simulink model "TP03"  (R2023a)
settings: Solver=ode45  StartTime=0.0  StopTime=2  FixedStep=5  RelTol=1e-3
undefined symbols (not defined in the file): DiscIntNeverNeededParam, K, ue, x0, xe
libraries: simulink x1
settings Model: Creator=pmt1554  LastModifiedBy=pmt1554

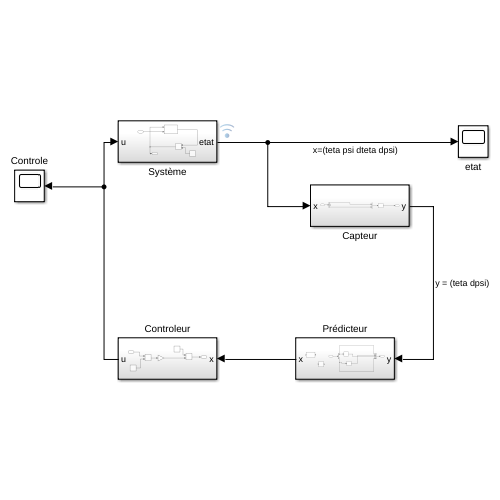
[thumbnail: Simulink's stored preview of the top-level diagram]
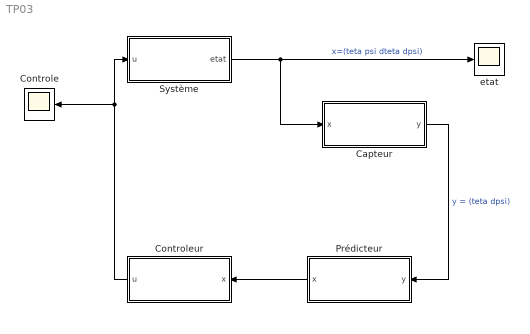
== system TP03 ==
  Capteur : Subsystem
  Controle : Scope
  Controleur : Subsystem
  Prédicteur : Subsystem
  Système : Subsystem
  etat : Scope
  wires:
  Système/1(etat) -> Capteur/1(x), etat/1  "x=(teta psi dteta dpsi)"
  Controleur/1(u) -> Système/1(u), Controle/1
  Capteur/1(y) -> Prédicteur/1(y)  "y = (teta dpsi)"
  Prédicteur/1(x) -> Controleur/1(x)

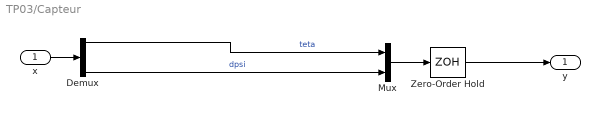
== system TP03/Capteur ==
  x : Inport
  Demux : Demux
  Mux : Mux  Inputs=2
  Zero-Order Hold : ZeroOrderHold  SampleTime=0.001
  y : Outport
  wires:
  x/1 -> Demux/1
  Mux/1 -> Zero-Order Hold/1
  Demux/1 -> Mux/1  "teta"
  Demux/4 -> Mux/2  "dpsi"
  Zero-Order Hold/1 -> y/1

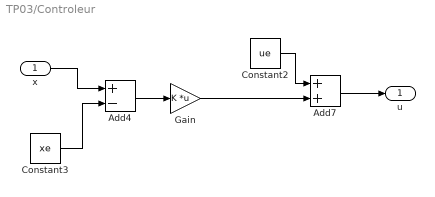
== system TP03/Controleur ==
  x : Inport
  Add4 : Sum  Inputs=+-
  Add7 : Sum
  Constant2 : Constant  Value=ue
  Constant3 : Constant  Value=xe
  Gain : Gain  Gain=K  Multiplication=Matrix(K*u)
  u : Outport
  wires:
  Constant2/1 -> Add7/1
  Add7/1 -> u/1
  x/1 -> Add4/1
  Constant3/1 -> Add4/2
  Add4/1 -> Gain/1
  Gain/1 -> Add7/2

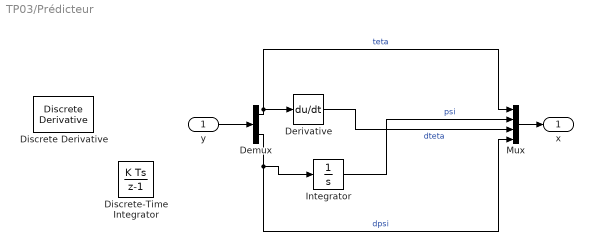
== system TP03/Prédicteur ==
  y : Inport
  Demux : Demux  Outputs=2
  Derivative : Derivative
  Discrete Derivative : simulink/Discrete/Discrete Derivative  gainval=1.0  ICPrevScaledInput=0.0  OutMin=[]  OutMax=[]  OutDataType=fixdt(1, 16)  OutScaling=2^-10  DoSatur=off
  Discrete-Time Integrator : DiscreteIntegrator  InitialCondition=x0(2)  SampleTime=-1  ICPrevOutput=DiscIntNeverNeededParam  ICPrevScaledInput=DiscIntNeverNeededParam
  Integrator : Integrator  InitialCondition=x0(2)
  Mux : Mux
  x : Outport
  wires:
  y/1 -> Demux/1
  Mux/1 -> x/1
  Demux/1 -> Derivative/1, Mux/1  "teta"
  Demux/2 -> Integrator/1, Mux/4  "dpsi"
  Integrator/1 -> Mux/2  "psi"
  Derivative/1 -> Mux/3  "dteta"

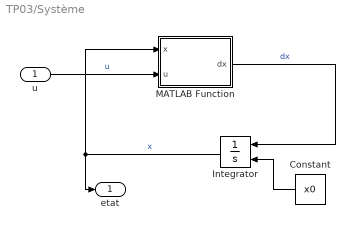
== system TP03/Système ==
  u : Inport
  Constant : Constant  Value=x0
  Integrator : Integrator  InitialConditionSource=external
  MATLAB Function : MATLAB Function  TreatAsAtomicUnit=on
  etat : Outport
  wires:
  MATLAB Function/1(dx) -> Integrator/1  "dx"
  Integrator/1 -> MATLAB Function/1(x), etat/1  "x"
  u/1 -> MATLAB Function/2(u)  "u"
  Constant/1 -> Integrator/2

== matlab function TP03/Système/MATLAB Function ==
  data: x input; u input; dx output
function dx    = fonction( x, u)
%   Dynamic equations of motion of the segway on an axis.
%   Inputs: - x = [theta psi dtheta dpsi]
%               theta: average angle of the wheels      [rad]
%               psi: body pitch angle                   [rad]
%               dtheta: average velocity of the wheels  [rad/s]
%               dpsi: body pitch velocity               [rad/s]
%          - u: DC motor voltage (same value for both motors) [V]

    % State
    psi = x(2);
    dtheta = x(3);
    dpsi = x(4);

    % Parameters
    
    g = 9.81;           % gravity acceleration [m/sec^2]
    m = 0.03;           % wheel weight [kg]
    R = 0.04;           % wheel radius [m]
    Jw = m*R^2/2;       % wheel inertia moment [kg*m^2]
    M = 0.6;            % body weight [kg]
    H = 0.144;          % body height [m]
    L = H/2;            % distance of the center of mass from the wheel axle [m]
    Jpsi = M*L^2/3;     % body pitch inertia [kgm^2]
    Jm = 1e-5;          % DC motor inertia moment [kgm^2]
    Rm = 6.69;          % DC motor resistance [Ohm]
    Kb = 0.468;         % DC motor back EMF constant [Vsec/rad]
    Kt = 0.317;         % DC motor torque constant [Nm/A]
    n = 1;              % gear ratio
    fm = 0.0022;        % friction coefficient between body and DC motor
    fw = 0;             % friction coefficient between wheel and floor
    
    % Equations of motion
    c1 = (2*m+M)*R^2 + 2*Jw + 2*n^2*Jm;
    c2 = M*L*R*cos(psi) - 2*n^2*Jm;
    c3 = -M*L*R*dpsi^2*sin(psi);
    c4 = M*L^2 + Jpsi + 2*n^2*Jm;
    c5 = -M*g*L*sin(psi);

    alpha = Kt/Rm;
    beta = Kt*Kb/Rm + fm;

    Ftheta = alpha*(2*u) - 2*(beta+fw)*dtheta + 2*beta*dpsi;
    Fpsi = -alpha*(2*u) + 2*beta*dtheta - 2*beta*dpsi;

    ddtheta = (c4*c3 - c2*c5 + c4*Ftheta - c2*Fpsi)/(c4*c1 - c2^2);
    ddpsi = (Fpsi- c2*ddtheta - c5)/c4;
    dx = [dtheta dpsi ddtheta ddpsi]';

end
